simulink model "my_sim"  (R2022a)
settings: Solver=VariableStepAuto  StartTime=0.0  StopTime=10.0  RelTol=1e-3
libraries: cstblocks x2
settings Model: Creator=apple  LastModifiedBy=apple

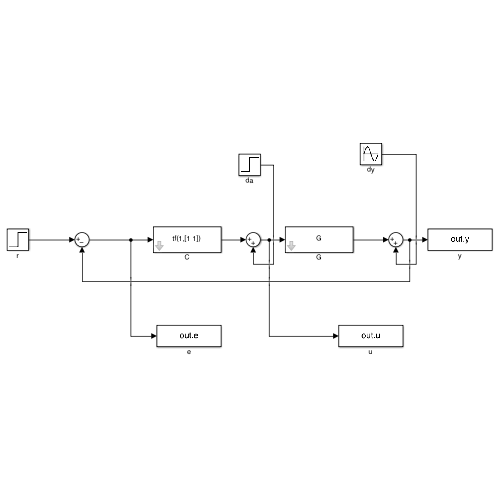
[thumbnail: Simulink's stored preview of the top-level diagram]
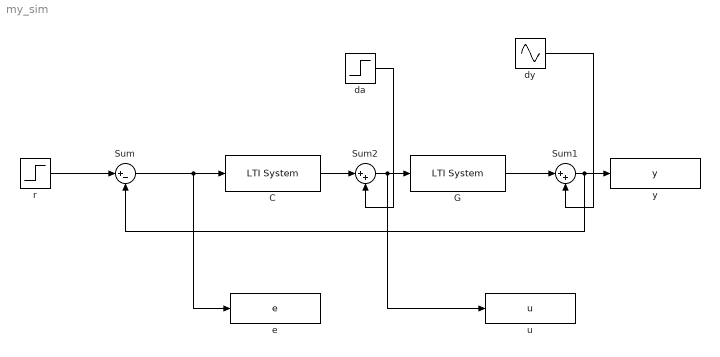
== system my_sim ==
  C : cstblocks/LTI System  sys=tf(1,[1 1])  IC=[]
  G : cstblocks/LTI System  sys=G  IC=[]
  Sum : Sum  Inputs=|+-
  Sum1 : Sum  Inputs=|++
  Sum2 : Sum  Inputs=|++
  da : Step  Time=0  SampleTime=0
  dy : Sin  SampleTime=0
  e : ToWorkspace  VariableName=e  SaveFormat=Timeseries  SampleTime=-1
  r : Step  Time=0  After=0  SampleTime=0
  u : ToWorkspace  VariableName=u  SaveFormat=Timeseries  SampleTime=-1
  y : ToWorkspace  VariableName=y  SaveFormat=Timeseries  SampleTime=-1
  wires:
  C/1 -> Sum2/1
  da/1 -> Sum2/2
  Sum2/1 -> u/1, G/1
  G/1 -> Sum1/1
  Sum1/1 -> y/1, Sum/2
  dy/1 -> Sum1/2
  r/1 -> Sum/1
  Sum/1 -> e/1, C/1
